simulink model "franka_placement_task_2019b"  (R2019b)
settings: Solver=FixedStepAuto  StartTime=0.0  StopTime=20  FixedStep=0.01  RelTol=1e-3
values from neighbouring files (symbols this model uses):
  a0 = 0.99    [init.m]
  berta = 0.98    [init.m]
  csi = 1    [init.m]
  e_max = 0.01    [init.m]
  F_int_max = 5    [init.m]
  F_max = 2    [init.m]
  g = 9.81    [init.m]
  k_can = 500    [init.m]
  k_shelf = k_table    (= 10000)    [init.m]
  k_table = 10000    [init.m]
  k_wall = k_table    (= 10000)    [init.m]
  l_can = 0.1    [init.m]
  M = 1    [init.m]
  mass = 1    [init.m]
  mass_can = 0.5    [init.m]
  q_max = q_max - deg2rad([0 0 0 10 0 5 0])    [init.m]
  q_min = q_min + deg2rad([0 0 0 10 0 5 0])    [init.m]
  y_can = 0.2    [init.m]
  y_wall = -0.3    [init.m]
  z_shelf = 0.3+0.043    (= 0.343)    [init.m]
  z_table = 0+0.043    (= 0.043)    [init.m]
(part 2 of 2)

== matlab function franka_placement_task_2019b/direct kinematics ==
  data: q_dot input double; q input double; z output double; dz output double; or output
function [z,dz,or] = fcn(q_dot,q)
% persistent dh_c
% if isempty(dh_c)
%     dh_c = Load_Franka_DH();
% end
[DH, Conv] = Load_Franka_DH();
z = zeros(3,1);
%z = get_pos(q);

[p,R] = DirectKinematic(DH,[q;0],Conv);
z = p;
phi = atan2(R(2,1),R(1,1));
teta = atan2(-R(3,1),sqrt(R(3,2)^2 + R(3,3)^2)); 
psi = atan2(R(3,2),R(3,3));
or = [phi teta psi]';

Ja = zeros(3,7);
Ja = get_Jacobianoa(q);

dz = zeros(3,1);
dz = Ja(1:3,1:7)*q_dot;

end

== matlab function franka_placement_task_2019b/PLANNER1/KZ_GENERATOR ==
  settings: updateMethod=DISCRETE  sampleTime=Ts
  data: k output; F_ext input; z input; z_des input; int input; comp input; e_max parameter; F_max parameter; F_int_max parameter
function k = fcn(F_ext, z, z_des, int, comp, e_max, F_max, F_int_max)
%% Description
% Set the K coefficient for a variable impedance controller based on a
% desired trajectory

%% Outputs
% k             stiffness

%% Inputs
% F_ext         measured external force
% z_des         desired trajectory
% z             current position
% int, comp     booleans for the interaction and compensation phase

%% Parameters
% F_int_max     desired interaction force
% F_max         nominal disturbance forces
% e_max         maximum steady-state error

%% persistent initialization
persistent ki kc F_comp int_prec comp_prec z_int z_int_dir 
if isempty(ki)
   ki = F_max/e_max;        % k obtained from interaction
end
if isempty(F_comp)
   F_comp = 0;              % weight to compensate
end
if isempty(kc)
      kc = F_max/e_max;     % k obtained from compensation
end
if isempty(z_int) 
    z_int = 1000;       % obstacle(or interaction) position
end
if isempty(z_int_dir) 
    z_int_dir = 0;          % prohibited direction due to the obstacle
end
if isempty(int_prec)
    int_prec = 0;           % previous values of int
end
if isempty(comp_prec)
    comp_prec = 0;          % previous values od comp
end

%% INTERACTION
% set ki in order to match a desired interaction force with the
% envirorment, and store interaction's position when detected
% X axes
if int == 1
    % detection of an interaction 
    if abs(F_ext-F_comp) > F_max
        if z_int == 1000                     % z_int has not been set yet
            z_int = z;
            z_int_dir = -sign(F_ext-F_comp);
        end
    end
    % setting of ki
    if abs(F_ext-F_comp) > F_int_max 
        % if interaction force is higher than threshold
        if ki*abs(z-z_des) > F_int_max
            ktemp_x = F_int_max/abs(z-z_des);
            if ktemp_x < ki                % ki needs to be only decreased
                ki = ktemp_x;
            end
        end
    end
end

%% COMPENSATION
% set kc in order to compensate the effect of the weight of the object,
% and store it
% X axes
if comp == 1
    % compensation detection
    if z_int == 1000                     % z_int not set before
       if abs(F_ext)/kc > e_max         
            kc = abs(F_ext)/e_max;
            F_comp = F_ext;
       end
    else 
        if z_int_dir == 1                % obstacle in above
            if z < z_int
                if abs(F_ext)/kc > e_max 
                    kc = abs(F_ext)/e_max;
                    F_comp = F_ext;
                end
            end
        else                                % obstacle is below
            if z > z_int
                if abs(F_ext)/kc > e_max
                    kc = abs(F_ext)/e_max;
                    F_comp = F_ext;
                end
            end
        end 
   end
end

%% reset to default values when comp or int shifts to zero
if comp==0 && comp_prec==1
    kc = F_max/e_max;
    F_comp = 0;
end
if int==0 && int_prec==1
    ki = F_max/e_max;
end

%% from int to comp and vice versa
if int==1 && int_prec==0
    if comp_prec == 1
        ki = kc;
    end
    z_int=1000;
    z_int_dir=0;
end
if comp == 1 && comp_prec==0
    if int_prec == 1
        kc = ki;
    end
end

% update to last booleans
int_prec = int;
comp_prec = comp;


%% Selection of Final Values of D-K
% default values
k = abs(F_max)/e_max;

% compensation
if comp == 1
    k = kc;
end

% both compensation and interaction are activated
% if "away" from obstacle set k = kc else ki
if int == 1
    k = ki;
    if comp == 1
        if z_int == 1000
            k = kc;                       % obstacle not reached
        else
            if z_int_dir == 1
                if z_des < z_int
                    k = kc;               % obstacle reached but "going away"
                end
            else
                if z_des > z_int
                    k = kc;               % obstacle reached but "going away"
                end
            end
        end
    else
        if z_int == 1000
            k = F_max/e_max;            % restore to default
        else
            if z_int_dir == 1
                if z_des < z_int
                    k = F_max/e_max;    % restore because "going away"
                end
            else
                if z_des > z_int
                    k = F_max/e_max;    % restore because "going away"
                end
            end
        end
    end
end

end

== matlab function franka_placement_task_2019b/direct kinematics1 ==
  data: q_dot input double; q input double; z output double; dz output double; or output
function [z,dz,or] = fcn(q_dot,q)
coder.extrinsic('get_Ja');
% persistent dh_c
% if isempty(dh_c)
%     dh_c = Load_Franka_DH();
% end
[DH, Conv] = Load_Franka_DH();
z = zeros(3,1);
%z = get_pos(q);

[p,R] = DirectKinematic(DH,[q;0],Conv);
z = p;
phi = atan2(R(2,1),R(1,1));
teta = atan2(-R(3,1),sqrt(R(3,2)^2 + R(3,3)^2)); 
psi = atan2(R(3,2),R(3,3));
or = [phi teta psi]';

Ja = zeros(6,7);
Ja = get_Ja(q);

dz = zeros(3,1);
dz = Ja(1:3,1:7)*q_dot;

end

== matlab function franka_placement_task_2019b/PLANNER/KD_INTERPOLATOR  ==
  settings: updateMethod=DISCRETE  sampleTime=Ts
  data: time input; K output; kx_f input; ky_f input; kz_f input; D output; e_max parameter; F_max parameter; M parameter; berta parameter; a0 parameter; mass parameter; csi parameter
function [K,D] = fcn(time, kx_f, ky_f, kz_f, e_max, F_max, M, berta, a0, mass, csi)
%% Description
% Interpolate K in order to guarantee stability

%% Outputs
% K             Stiffness matrix
% D             Damping matrix

%% Inputs
% kx_f, ky, f   desired values of K

%% Parameters
% F_max         nominal disturbance forces
% e_max         maximum steady-state error
% M             virtual mass
% berta, a0     parameters for the computation of stability conditions
% mass          virtual mass

%% persistent initialization
persistent kx ky kz time_prec
if isempty(time_prec)
    time_prec = 0;              % previous simulation time
end
if isempty(kx)
   kx = F_max/e_max;         % last value of k
end
if isempty(ky)
   ky = F_max/e_max;
end
if isempty(kz)
   kz = F_max/e_max;
end

% set k from desired one 
if kx_f <= kx       
    kx = kx_f;
else 
    % increese k in accordance with the stability conditions
    kx_i = kx;
    k_dotx = berta*(4*a0*sqrt(kx_i/mass)*(kx_i)^(3/2))/(sqrt(kx_i) + 2*a0*csi*sqrt(kx_i));
    k_tempx = kx_i + k_dotx*(time -time_prec);
    if k_tempx > kx_f
        kx = kx_f;
    else
        kx = k_tempx;
    end
end

% Y axes, same as X axes
if ky_f <= ky
    ky = ky_f;
else 
    ky_i = ky;
    k_doty = berta*(4*a0*sqrt(ky_i/mass)*(ky_i)^(3/2))/(sqrt(ky_i) + 2*a0*csi*sqrt(ky_i));
    k_tempy = ky_i + k_doty*(time -time_prec);
    if k_tempy > ky_f
        ky = ky_f;
    else
        ky = k_tempy;
    end
end

% Z axes, same as other axes
if kz_f <= kz
    kz = kz_f;
else 
    kz_i = kz;
    k_dotz = berta*(4*a0*sqrt(kz_i/mass)*(kz_i)^(3/2))/(sqrt(kz_i) + 2*a0*csi*sqrt(kz_i));
    k_tempz = kz_i + k_dotz*(time -time_prec);
    if k_tempz > kz_f
        kz = kz_f;
    else
        kz = k_tempz;
    end
end

time_prec = time;

% damping computation, critically damped condition
dx = sqrt(4*kx*M);
dy = sqrt(4*ky*M);
dz = sqrt(4*kz*M);

%% Final impedance matrices
D = diag([dx, dy, dz]);
K = diag([kx, ky, kz]);

end

== matlab function franka_placement_task_2019b/PLANNER/KX_GENERATOR ==
  settings: updateMethod=DISCRETE  sampleTime=Ts
  data: k output; F_ext input; z input; z_des input; int input; comp input; e_max parameter; F_max parameter; F_int_max parameter
function k = fcn(F_ext, z, z_des, int, comp, e_max, F_max, F_int_max)
%% Description
% Set the K coefficient for a variable impedance controller based on a
% desired trajectory

%% Outputs
% k             stiffness

%% Inputs
% F_ext         measured external force
% z_des         desired trajectory
% z             current position
% int, comp     booleans for the interaction and compensation phase

%% Parameters
% F_int_max     desired interaction force
% F_max         nominal disturbance forces
% e_max         maximum steady-state error

%% persistent initialization
persistent ki kc F_comp int_prec comp_prec z_int z_int_dir 
if isempty(ki)
   ki = F_max/e_max;        % k obtained from interaction
end
if isempty(F_comp)
   F_comp = 0;              % weight to compensate
end
if isempty(kc)
      kc = F_max/e_max;     % k obtained from compensation
end
if isempty(z_int) 
    z_int = 1000;       % obstacle(or interaction) position
end
if isempty(z_int_dir) 
    z_int_dir = 0;          % prohibited direction due to the obstacle
end
if isempty(int_prec)
    int_prec = 0;           % previous values of int
end
if isempty(comp_prec)
    comp_prec = 0;          % previous values od comp
end

%% INTERACTION
% set ki in order to match a desired interaction force with the
% envirorment, and store interaction's position when detected
% X axes
if int == 1
    % detection of an interaction 
    if abs(F_ext-F_comp) > F_max
        if z_int == 1000                     % z_int has not been set yet
            z_int = z;
            z_int_dir = -sign(F_ext-F_comp);
        end
    end
    % setting of ki
    if abs(F_ext-F_comp) > F_int_max 
        % if interaction force is higher than threshold
        if ki*abs(z-z_des) > F_int_max
            ktemp_x = F_int_max/abs(z-z_des);
            if ktemp_x < ki                % ki needs to be only decreased
                ki = ktemp_x;
            end
        end
    end
end

%% COMPENSATION
% set kc in order to compensate the effect of the weight of the object,
% and store it
% X axes
if comp == 1
    % compensation detection
    if z_int == 1000                     % z_int not set before
       if abs(F_ext)/kc > e_max         
            kc = abs(F_ext)/e_max;
            F_comp = F_ext;
       end
    else 
        if z_int_dir == 1                % obstacle in above
            if z < z_int
                if abs(F_ext)/kc > e_max 
                    kc = abs(F_ext)/e_max;
                    F_comp = F_ext;
                end
            end
        else                                % obstacle is below
            if z > z_int
                if abs(F_ext)/kc > e_max
                    kc = abs(F_ext)/e_max;
                    F_comp = F_ext;
                end
            end
        end 
   end
end

%% reset to default values when comp or int shifts to zero
if comp==0 && comp_prec==1
    kc = F_max/e_max;
    F_comp = 0;
end
if int==0 && int_prec==1
    ki = F_max/e_max;
end

%% from int to comp and vice versa
if int==1 && int_prec==0
    if comp_prec == 1
        ki = kc;
    end
    z_int=1000;
    z_int_dir=0;
end
if comp == 1 && comp_prec==0
    if int_prec == 1
        kc = ki;
    end
end

% update to last booleans
int_prec = int;
comp_prec = comp;


%% Selection of Final Values of D-K
% default values
k = abs(F_max)/e_max;

% compensation
if comp == 1
    k = kc;
end

% both compensation and interaction are activated
% if "away" from obstacle set k = kc else ki
if int == 1
    k = ki;
    if comp == 1
        if z_int == 1000
            k = kc;                       % obstacle not reached
        else
            if z_int_dir == 1
                if z_des < z_int
                    k = kc;               % obstacle reached but "going away"
                end
            else
                if z_des > z_int
                    k = kc;               % obstacle reached but "going away"
                end
            end
        end
    else
        if z_int == 1000
            k = F_max/e_max;            % restore to default
        else
            if z_int_dir == 1
                if z_des < z_int
                    k = F_max/e_max;    % restore because "going away"
                end
            else
                if z_des > z_int
                    k = F_max/e_max;    % restore because "going away"
                end
            end
        end
    end
end

end

== matlab function franka_placement_task_2019b/TRAJECTORY/INTERPOLATOR ==
  data: xi input; z_des output; xf input; tf input; t input; v input; alpha input; dz_des output; ddz_des output
function [z_des, dz_des, ddz_des] = fcn(xi, xf, tf, t, v, alpha)

ta = alpha*tf; 
xa = (1/2)*v*ta;

if t >= 0 && t < ta
    ddz_des = v./ta;
    dz_des = ddz_des*t;
    z_des = xi + (1/2)*ddz_des*t^2;
elseif t >= ta && t < (tf-ta)
    ddz_des = [0; 0; 0]; 
    dz_des = v; 
    z_des = xi + xa + dz_des*(t-ta);
elseif t >= (tf- ta) && t < tf
    ddz_des = -v./ta;
    dz_des = v + ddz_des*(t - (tf-ta));
    z_des = xi + xa + v*(tf-2*ta) + v*(t-(tf-ta)) + (1/2)*ddz_des*(t-(tf-ta))^2;
else 
    ddz_des = [0; 0; 0];
    dz_des = [0; 0; 0];
    z_des = xf;
end

end

== matlab function franka_placement_task_2019b/FRANKA_Model_Joint_Space1/GRAVITY ==
  data: q input; G output double
function G = fcn(q)

G = zeros(7,1);
G = get_GravityVector(q);

end

== matlab function franka_placement_task_2019b/FRANKA_Model_Joint_Space1/Joint Friction1 ==
  data: q_dot input; tau_f output
function tau_f = fcn(q_dot)
D=eye(7)*1;
tau_f = -D*q_dot;

end

== matlab function franka_placement_task_2019b/FRANKA_Model_Joint_Space1/Joint Friction ==
  data: q_dot input; tau_f output
function tau_f = fcn(q_dot)

tau_f = get_FrictionTorque(q_dot);

end

== matlab function franka_placement_task_2019b/M_D_S5/DAMPER ==
  data: dx input; y output; D input
function y = fcn(dx, D)
y = - D*dx;
end

== matlab function franka_placement_task_2019b/M_D_S5/MASS^-1 ==
  data: M input; ddx output; F_tot input
function ddx = fcn(M,F_tot)
ddx = (M^-1)*F_tot;


end

== matlab function franka_placement_task_2019b/M_D_S5/SPRING ==
  data: x input; tau output; K input
function tau = fcn(x, K)
tau= -K*x;
end

== matlab function franka_placement_task_2019b/FRANKA_Model_Joint_Space1/MASS^-1 ==
  data: q input; ddq output; F_tot input double
function ddq = fcn(q,F_tot)

B = zeros(7,7);
B = get_MassMatrix(q);

ddq = B\F_tot;                      % Ftot*M^-1

end

== matlab function franka_placement_task_2019b/FRANKA_Model_Joint_Space1/MATLAB Function ==
  data: F input; F_ext output double; q input
function F_ext = fcn(F,q)

Ja = zeros(6,7);
Ja = get_Jacobianoa(q);

F_ext = zeros(7,1);
F_ext = (Ja')*F;

end

== matlab function franka_placement_task_2019b/MATLAB Function ==
  data: K output; D output
function [K, D] = fcn()
K = zeros(6,6);
K(1:3,1:3) = diag([1000 1000 1000]); %Klin
K(4:6,4:6) = diag ([300 300 300]); %Kor
D = zeros(6,6);
D(1:3,1:3) = diag([2*sqrt(1000) 2*sqrt(1000) 2*sqrt(1000)]);
D(4:6,4:6) = diag([2*sqrt(300) 2*sqrt(300) 2*sqrt(300)]);

end

== matlab function franka_placement_task_2019b/CONTROLLER1 ==
  data: F_ext input; Km input; Dm input; or_des input; zdes input; tau output double; dzdes input; ddzdes input; q input; q_dot input; M parameter
function tau = fcn(F_ext, Km, Dm, or_des, zdes, dzdes, ddzdes, q, q_dot, M)
coder.extrinsic('get_MassMatrix','get_Ja_dot','get_Ja','get_GravityVector','get_FrictionTorque','get_CoriolisMatrix')
coder.extrinsic('wrapToPi');
% dz = zeros(2,1);
% z = zeros(2,1);
B = zeros(7,7);
S = zeros(7,7);
G = zeros(7,1);
Ja = zeros(6,7);
Ja_dot = zeros(6,7);
tau_fric = zeros(7,1);
Bm = eye(6)*M;
Ja = get_Ja(q);
Ja(isnan(Ja)) = 1;
% cond_Ja = cond(Ja)
Ja_dot = get_Ja_dot(q,q_dot);
Ja_dot(isnan(Ja_dot)) = 1;

% cond_Ja_dot = cond(Ja_dot)

%% Computation of end-effector's position and orientation 
[DH, Conv] = Load_Franka_DH();
[p,R] = DirectKinematic(DH,[q;0],Conv);
z = zeros(3,1);
%z = get_pos(q);
z = p;
dz = Ja(1:3,1:7)*q_dot;
phi = atan2(R(2,1),R(1,1));
teta = atan2(-R(3,1),sqrt(R(3,2)^2 + R(3,3)^2)); 
psi = atan2(R(3,2),R(3,3));
or = [phi teta psi]';

% pseudoinverse
B = get_MassMatrix(q);
B_inv = inv(B);
B_inv(isnan(B_inv)) = 1;
Ja_inv = B_inv*(Ja')*inv(Ja*B_inv*Ja');
Ja_inv(isnan(Ja_inv)) = 1;

% cond_Ja_inv = cond(Ja_inv)
% cond_B = cond(B)


% Matrices
S = get_CoriolisMatrix(q,q_dot);
tau_fric = get_FrictionTorque(q_dot);
G = get_GravityVector(q);
I = eye(6);

% Impedance controller (De Luca)
%{
Bx = (Ja_inv')* B * Ja_inv;
tau = B*Ja_inv*(ddzdes - Ja_dot*q_dot + ...
    inv(Bm)*(Dm*(dzdes - dz) + Km*(zdes- z))) + S*q_dot + tau_fric + G + ...
    (Ja')*(Bx*inv(Bm) - I)*F_ext;
%}
% Impedance controller (Albu Shaffer)
L = inv(Ja * B_inv * Ja');
L(isnan(L)) = 1;
% cond_L = cond(L)
e_pos = (z - zdes);
e_pos_dot = (dz - dzdes);
%e_or = (or - or_des); 
e_or = zeros(3,1);
e_or = wrapToPi(or-or_des);
e_or_dot = Ja(4:6,1:7)*q_dot;
e = [e_pos; e_or];
e_dot = [e_pos_dot; e_or_dot];                                                                   
a_des = [ddzdes; zeros(3,1)];
F_tau = L*a_des - L*inv(Bm)*(Dm*e_dot + Km*e) + (L*inv(Bm) - I)*F_ext - L*Ja_dot*q_dot;
tau = (Ja')*F_tau + S*q_dot + tau_fric + G;

end

== matlab function franka_placement_task_2019b/FRANKA_Model_Joint_Space2/CORIOLIS ==
  data: q input; Fc output double; q_dot input
function Fc = fcn(q,q_dot)
coder.extrinsic('get_CoriolisMatrix');
C = zeros(7,7);
C = get_CoriolisMatrix(q,q_dot);

Fc = C*q_dot;

end

== matlab function franka_placement_task_2019b/FRANKA_Model_Joint_Space2/GRAVITY ==
  data: q input; G output double
function G = fcn(q)
coder.extrinsic('get_GravityVector');
G = zeros(7,1);
G = get_GravityVector(q);

end

== matlab function franka_placement_task_2019b/FRANKA_Model_Joint_Space2/Joint Friction ==
  data: q_dot input; tau_f output
function tau_f = fcn(q_dot)
coder.extrinsic('get_FrictionTorque');
tau_f = zeros(7,1);
tau_f = get_FrictionTorque(q_dot);

end

== matlab function franka_placement_task_2019b/FRANKA_Model_Joint_Space2/Joint Friction1 ==
  data: q_dot input; tau_f output
function tau_f = fcn(q_dot)
D=eye(7)*1;
tau_f = -D*q_dot;

end

== matlab function franka_placement_task_2019b/FRANKA_Model_Joint_Space2/MASS^-1 ==
  data: q input; ddq output; F_tot input double
function ddq = fcn(q,F_tot)
coder.extrinsic('get_MassMatrix');
B = zeros(7,7);
B = get_MassMatrix(q);

% ddq = B\F_tot;     % Ftot*M^-1

B_inv = inv(B);
B_inv(isnan(B_inv)) = 1;
ddq = B_inv*F_tot;

% B_modello = cond(B)

end

== matlab function franka_placement_task_2019b/FRANKA_Model_Joint_Space2/MATLAB Function ==
  data: F input; F_ext output double; q input
function F_ext = fcn(F,q)
coder.extrinsic('get_Ja');
Ja = zeros(6,7);
Ja = get_Ja(q);

F_ext = zeros(7,1);
F_ext = (Ja')*F;

end

== matlab function franka_placement_task_2019b/F_ext4 ==
  data: z input; F_ext output; grasping input; mass_can parameter; g parameter; phase input; y_can parameter; z_table parameter; k_can parameter; k_table parameter; l_can parameter; y_wall parameter; z_shelf parameter; k_wall parameter; k_shelf parameter
function F_ext = fcn(z, grasping, mass_can, g, phase, y_can, z_table, k_can, k_table, l_can, y_wall, z_shelf, k_wall, k_shelf) 

% hypothesis: table reaction force with elastic behaviour
F_ext = zeros(3,1);
F_ext(1) = 0;
if phase == 1
    % if contact is happened with can
    if grasping == 0
        if z(2) < y_can
            F_ext(2) = -k_can*(z(2) - y_can);    
        end
        if z(3) < z_table
            F_ext(3) = -k_table*(z(3) - z_table);
        end
    else 
        if z(3) < z_table
            F_ext(3) = -k_table*(z(3)-z_table);       
        else 
            if (abs(k_table*(z(3)-z_table)) < abs(mass_can*g))
                F_ext(3) = - k_table*(z(3)-z_table); 
            else 
                F_ext(3) = - mass_can*g;
            end    
        end
    end
elseif phase == 2
    if z(2) < y_wall + l_can
        F_ext(2) = -k_wall*(z(2) - (l_can + y_wall));
    end
    if z(3) < z_shelf
        F_ext(3) = -k_shelf*(z(3) - z_shelf);
    else 
        if (abs(k_shelf*(z(3)-z_shelf)) < abs(mass_can*g))
            F_ext(3) = - k_shelf*(z(3)-z_shelf); 
        else 
            F_ext(3) = - mass_can*g;
        end 
    end
else
    if z(2) < y_wall + l_can
        F_ext(2) = -k_wall*(z(2) - (l_can + y_wall));
    end
    if z(3) < z_shelf
        F_ext(3) = -k_shelf*(z(3) - z_shelf);
    end
end

== matlab function franka_placement_task_2019b/PLANNER2/KY_GENERATOR ==
  settings: updateMethod=DISCRETE  sampleTime=Ts
  data: k output; F_ext input; z input; z_des input; dz_des input; int input; comp input; e_max parameter; F_max parameter; F_int_max parameter
function k = fcn(F_ext, z, z_des, dz_des, int, comp, e_max, F_max, F_int_max)
%% Description
% Set the K coefficient for a variable impedance controller based on a
% desired trajectory

%% Outputs
% k             stiffness

%% Inputs
% F_ext         measured external force
% z_des         desired trajectory
% z             current position
% int, comp     booleans for the interaction and compensation phase

%% Parameters
% F_int_max     desired interaction force
% F_max         nominal disturbance forces
% e_max         maximum steady-state error

%% persistent initialization
persistent ki kc F_comp int_prec comp_prec z_int z_int_dir set_F_comp
if isempty(ki)
   ki = F_max/e_max;        % k obtained from interaction
end
if isempty(F_comp)
   F_comp = 0;              % weight to compensate
end
if isempty(kc)
      kc = F_max/e_max;     % k obtained from compensation
end
if isempty(z_int) 
    z_int = 1000;       % obstacle(or interaction) position
end
if isempty(z_int_dir) 
    z_int_dir = 0;          % prohibited direction due to the obstacle
end
if isempty(int_prec)
    int_prec = 0;           % previous values of int
end
if isempty(comp_prec)
    comp_prec = 0;          % previous values od comp
end
if isempty(set_F_comp)
    set_F_comp = 1;
end
%% INTERACTION
% set ki in order to match a desired interaction force with the
% envirorment, and store interaction's position when detected
% X axes
if int == 1
    % detection of an interaction 
    if abs(F_ext-F_comp) > F_max
        if z_int == 1000                     % z_int has not been set yet
            z_int = z;
            z_int_dir = -sign(F_ext-F_comp);
            set_F_comp = 0; 
        end
    end
    % setting of ki
    if abs(F_ext-F_comp) > F_int_max 
        % if interaction force is higher than threshold
        if ki*abs(z-z_des) > F_int_max
            ktemp_x = F_int_max/abs(z-z_des);
            if ktemp_x < ki                % ki needs to be only decreased
                ki = ktemp_x;
            end
        end
    end
end

%% COMPENSATION
% set kc in order to compensate the effect of the weight of the object,
% and store it
% X axes
if comp == 1
    % compensation detection
    if z_int == 1000                     % z_int not set before
        if abs(F_ext)/kc > e_max         
            kc = abs(F_ext)/e_max;
            if set_F_comp > 0.1
                F_comp = F_ext;
            end
        end
    else 
        if z_int_dir == 1                % obstacle in above
            if z < z_int
                if abs(F_ext)/kc > e_max 
                    kc = abs(F_ext)/e_max;
                    if set_F_comp > 0.1
                        F_comp = F_ext;
                    end
                end
            end
        else                                % obstacle is below
            if z > z_int
                if abs(F_ext)/kc > e_max
                    kc = abs(F_ext)/e_max;
                    if set_F_comp > 0.1
                        F_comp = F_ext;
                    end
                end
            end
        end 
   end
end

%% reset to default values when comp or int shifts to zero
if comp==0 && comp_prec==1
    kc = F_max/e_max;
    F_comp = 0;
    set_F_comp = 0;
end
if int==0 && int_prec==1
    ki = F_max/e_max;
end

%% from int to comp and vice versa
if int==1 && int_prec==0
    if comp_prec == 1
        ki = kc;
    end
    z_int=1000;
    z_int_dir=0;
end
if comp == 1 && comp_prec==0
    if int_prec == 1
        kc = ki;
    end
    set_F_comp = 1;
end

% update to last booleans
int_prec = int;
comp_prec = comp;


%% Selection of Final Values of D-K
% default values
k = abs(F_max)/e_max;

% compensation
if comp == 1
    k = kc;
end

% both compensation and interaction are activated
% if "away" from obstacle set k = kc else ki
if int == 1
    k = ki;
    if comp == 1
        if z_int == 1000
            k = kc;                       % obstacle not reached
        else
            if z_int_dir == 1
                if z_des < z_int
                    if sign(dz_des*z_int_dir) < 0
                        k = kc;               % obstacle reached but "going away"
                    end
                end
            else
                if z_des > z_int
                    if sign(dz_des*z_int_dir) < 0
                        k = kc;               % obstacle reached but "going away"
                    end
                end
            end
        end
    else
        if z_int == 1000
            k = F_max/e_max;            % restore to default
        else
            if z_int_dir == 1
                if z_des < z_int
                    k = F_max/e_max;    % restore because "going away"
                end
            else
                if z_des > z_int
                    k = F_max/e_max;    % restore because "going away"
                end
            end
        end
    end
end

end

== matlab function franka_placement_task_2019b/PLANNER2/KD_INTERPOLATOR  ==
  settings: updateMethod=DISCRETE  sampleTime=Ts
  data: time input; K output; kx_f input; ky_f input; kz_f input; D output; e_max parameter; F_max parameter; M parameter; berta parameter; a0 parameter; mass parameter; csi parameter; Kvis output; Dvis output
function [K,D,Kvis, Dvis] = fcn(time, kx_f, ky_f, kz_f, e_max, F_max, M, berta, a0, mass, csi)
%% Description
% Interpolate K in order to guarantee stability

%% Outputs
% K             Stiffness matrix
% D             Damping matrix

%% Inputs
% kx_f, ky, f   desired values of K

%% Parameters
% F_max         nominal disturbance forces
% e_max         maximum steady-state error
% M             virtual mass
% berta, a0     parameters for the computation of stability conditions
% mass          virtual mass

%% persistent initialization
persistent kx ky kz time_prec
if isempty(time_prec)
    time_prec = 0;              % previous simulation time
end
if isempty(kx)
   kx = F_max/e_max;         % last value of k
end
if isempty(ky)
   ky = F_max/e_max;
end
if isempty(kz)
   kz = F_max/e_max;
end

% set k from desired one 
if kx_f <= kx       
    kx = kx_f;
else 
    % increese k in accordance with the stability conditions
    kx_i = kx;
    k_dotx = berta*(4*a0*sqrt(kx_i/mass)*(kx_i)^(3/2))/(sqrt(kx_i) + 2*a0*csi*sqrt(kx_i));
    k_tempx = kx_i + k_dotx*(time -time_prec);
    if k_tempx > kx_f
        kx = kx_f;
    else
        kx = k_tempx;
    end
end

% Y axes, same as X axes
if ky_f <= ky
    ky = ky_f;
else 
    ky_i = ky;
    k_doty = berta*(4*a0*sqrt(ky_i/mass)*(ky_i)^(3/2))/(sqrt(ky_i) + 2*a0*csi*sqrt(ky_i));
    k_tempy = ky_i + k_doty*(time -time_prec);
    if k_tempy > ky_f
        ky = ky_f;
    else
        ky = k_tempy;
    end
end

% Z axes, same as other axes
if kz_f <= kz
    kz = kz_f;
else 
    kz_i = kz;
    k_dotz = berta*(4*a0*sqrt(kz_i/mass)*(kz_i)^(3/2))/(sqrt(kz_i) + 2*a0*csi*sqrt(kz_i));
    k_tempz = kz_i + k_dotz*(time -time_prec);
    if k_tempz > kz_f
        kz = kz_f;
    else
        kz = k_tempz;
    end
end

time_prec = time;

% damping computation, critically damped condition
dx = sqrt(4*kx*M);
dy = sqrt(4*ky*M);
dz = sqrt(4*kz*M);

%% Final impedance matrices
D = zeros(6,6);
K = zeros(6,6);
D(1:3,1:3) = diag([dx, dy, dz]);
D(4:6,4:6) = diag([2*sqrt(300) 2*sqrt(300) 2*sqrt(300)]); %rot damping
K(1:3,1:3) = diag([kx, ky, kz]);
K(4:6,4:6) = diag ([300 300 300]); %rot stiffness
Kvis = [kx; ky; kz];
Dvis = [dx; dy; dz];
end

== matlab function franka_placement_task_2019b/PLANNER2/KX_GENERATOR ==
  settings: updateMethod=DISCRETE  sampleTime=Ts
  data: k output; F_ext input; z input; z_des input; dz_des input; int input; comp input; e_max parameter; F_max parameter; F_int_max parameter
function k = fcn(F_ext, z, z_des, dz_des, int, comp, e_max, F_max, F_int_max)
%% Description
% Set the K coefficient for a variable impedance controller based on a
% desired trajectory

%% Outputs
% k             stiffness

%% Inputs
% F_ext         measured external force
% z_des         desired trajectory
% z             current position
% int, comp     booleans for the interaction and compensation phase

%% Parameters
% F_int_max     desired interaction force
% F_max         nominal disturbance forces
% e_max         maximum steady-state error

%% persistent initialization
persistent ki kc F_comp int_prec comp_prec z_int z_int_dir set_F_comp
if isempty(ki)
   ki = F_max/e_max;        % k obtained from interaction
end
if isempty(F_comp)
   F_comp = 0;              % weight to compensate
end
if isempty(kc)
      kc = F_max/e_max;     % k obtained from compensation
end
if isempty(z_int) 
    z_int = 1000;       % obstacle(or interaction) position
end
if isempty(z_int_dir) 
    z_int_dir = 0;          % prohibited direction due to the obstacle
end
if isempty(int_prec)
    int_prec = 0;           % previous values of int
end
if isempty(comp_prec)
    comp_prec = 0;          % previous values od comp
end
if isempty(set_F_comp)
    set_F_comp = 1;
end
%% INTERACTION
% set ki in order to match a desired interaction force with the
% envirorment, and store interaction's position when detected
% X axes
if int == 1
    % detection of an interaction 
    if abs(F_ext-F_comp) > F_max
        if z_int == 1000                     % z_int has not been set yet
            z_int = z;
            z_int_dir = -sign(F_ext-F_comp);
            set_F_comp = 0; 
        end
    end
    % setting of ki
    if abs(F_ext-F_comp) > F_int_max 
        % if interaction force is higher than threshold
        if ki*abs(z-z_des) > F_int_max
            ktemp_x = F_int_max/abs(z-z_des);
            if ktemp_x < ki                % ki needs to be only decreased
                ki = ktemp_x;
            end
        end
    end
end

%% COMPENSATION
% set kc in order to compensate the effect of the weight of the object,
% and store it
% X axes
if comp == 1
    % compensation detection
    if z_int == 1000                     % z_int not set before
        if abs(F_ext)/kc > e_max         
            kc = abs(F_ext)/e_max;
            if set_F_comp > 0.1
                F_comp = F_ext;
            end
        end
    else 
        if z_int_dir == 1                % obstacle in above
            if z < z_int
                if abs(F_ext)/kc > e_max 
                    kc = abs(F_ext)/e_max;
                    if set_F_comp > 0.1
                        F_comp = F_ext;
                    end
                end
            end
        else                                % obstacle is below
            if z > z_int
                if abs(F_ext)/kc > e_max
                    kc = abs(F_ext)/e_max;
                    if set_F_comp > 0.1
                        F_comp = F_ext;
                    end
                end
            end
        end 
   end
end

%% reset to default values when comp or int shifts to zero
if comp==0 && comp_prec==1
    kc = F_max/e_max;
    F_comp = 0;
    set_F_comp = 0;
end
if int==0 && int_prec==1
    ki = F_max/e_max;
end

%% from int to comp and vice versa
if int==1 && int_prec==0
    if comp_prec == 1
        ki = kc;
    end
    z_int=1000;
    z_int_dir=0;
end
if comp == 1 && comp_prec==0
    if int_prec == 1
        kc = ki;
    end
    set_F_comp = 1;
end

% update to last booleans
int_prec = int;
comp_prec = comp;


%% Selection of Final Values of D-K
% default values
k = abs(F_max)/e_max;

% compensation
if comp == 1
    k = kc;
end

% both compensation and interaction are activated
% if "away" from obstacle set k = kc else ki
if int == 1
    k = ki;
    if comp == 1
        if z_int == 1000
            k = kc;                       % obstacle not reached
        else
            if z_int_dir == 1
                if z_des < z_int
                    if sign(dz_des*z_int_dir) < 0
                        k = kc;               % obstacle reached but "going away"
                    end
                end
            else
                if z_des > z_int
                    if sign(dz_des*z_int_dir) < 0
                        k = kc;               % obstacle reached but "going away"
                    end
                end
            end
        end
    else
        if z_int == 1000
            k = F_max/e_max;            % restore to default
        else
            if z_int_dir == 1
                if z_des < z_int
                    k = F_max/e_max;    % restore because "going away"
                end
            else
                if z_des > z_int
                    k = F_max/e_max;    % restore because "going away"
                end
            end
        end
    end
end

end

== matlab function franka_placement_task_2019b/PLANNER2/KZ_GENERATOR ==
  settings: updateMethod=DISCRETE  sampleTime=Ts
  data: k output; F_ext input; z input; z_des input; dz_des input; int input; comp input; e_max parameter; F_max parameter; F_int_max parameter
function k = fcn(F_ext, z, z_des, dz_des, int, comp, e_max, F_max, F_int_max)
%% Description
% Set the K coefficient for a variable impedance controller based on a
% desired trajectory

%% Outputs
% k             stiffness

%% Inputs
% F_ext         measured external force
% z_des         desired trajectory
% z             current position
% int, comp     booleans for the interaction and compensation phase

%% Parameters
% F_int_max     desired interaction force
% F_max         nominal disturbance forces
% e_max         maximum steady-state error

%% persistent initialization
persistent ki kc F_comp int_prec comp_prec z_int z_int_dir set_F_comp
if isempty(ki)
   ki = F_max/e_max;        % k obtained from interaction
end
if isempty(F_comp)
   F_comp = 0;              % weight to compensate
end
if isempty(kc)
      kc = F_max/e_max;     % k obtained from compensation
end
if isempty(z_int) 
    z_int = 1000;       % obstacle(or interaction) position
end
if isempty(z_int_dir) 
    z_int_dir = 0;          % prohibited direction due to the obstacle
end
if isempty(int_prec)
    int_prec = 0;           % previous values of int
end
if isempty(comp_prec)
    comp_prec = 0;          % previous values od comp
end
if isempty(set_F_comp)
    set_F_comp = 1;
end
%% INTERACTION
% set ki in order to match a desired interaction force with the
% envirorment, and store interaction's position when detected
% X axes
if int == 1
    % detection of an interaction 
    if abs(F_ext-F_comp) > F_max
        if z_int == 1000                     % z_int has not been set yet
            z_int = z;
            z_int_dir = -sign(F_ext-F_comp);
            set_F_comp = 0; 
        end
    end
    % setting of ki
    if abs(F_ext-F_comp) > F_int_max 
        % if interaction force is higher than threshold
        if ki*abs(z-z_des) > F_int_max
            ktemp_x = F_int_max/abs(z-z_des);
            if ktemp_x < ki                % ki needs to be only decreased
                ki = ktemp_x;
            end
        end
    end
end

%% COMPENSATION
% set kc in order to compensate the effect of the weight of the object,
% and store it
% X axes
if comp == 1
    % compensation detection
    if z_int == 1000                     % z_int not set before
        if abs(F_ext)/kc > e_max         
            kc = abs(F_ext)/e_max;
            if set_F_comp > 0.1
                F_comp = F_ext;
            end
        end
    else 
        if z_int_dir == 1                % obstacle in above
            if z < z_int
                if abs(F_ext)/kc > e_max 
                    kc = abs(F_ext)/e_max;
                    if set_F_comp > 0.1
                        F_comp = F_ext;
                    end
                end
            end
        else                                % obstacle is below
            if z > z_int
                if abs(F_ext)/kc > e_max
                    kc = abs(F_ext)/e_max;
                    if set_F_comp > 0.1
                        F_comp = F_ext;
                    end
                end
            end
        end 
   end
end

%% reset to default values when comp or int shifts to zero
if comp==0 && comp_prec==1
    kc = F_max/e_max;
    F_comp = 0;
    set_F_comp = 0;
end
if int==0 && int_prec==1
    ki = F_max/e_max;
end

%% from int to comp and vice versa
if int==1 && int_prec==0
    if comp_prec == 1
        ki = kc;
    end
    z_int=1000;
    z_int_dir=0;
end
if comp == 1 && comp_prec==0
    if int_prec == 1
        kc = ki;
    end
    set_F_comp = 1;
end

% update to last booleans
int_prec = int;
comp_prec = comp;


%% Selection of Final Values of D-K
% default values
k = abs(F_max)/e_max;

% compensation
if comp == 1
    k = kc;
end

% both compensation and interaction are activated
% if "away" from obstacle set k = kc else ki
if int == 1
    k = ki;
    if comp == 1
        if z_int == 1000
            k = kc;                       % obstacle not reached
        else
            if z_int_dir == 1
                if z_des < z_int
                    if sign(dz_des*z_int_dir) < 0
                        k = kc;               % obstacle reached but "going away"
                    end
                end
            else
                if z_des > z_int
                    if sign(dz_des*z_int_dir) < 0
                        k = kc;               % obstacle reached but "going away"
                    end
                end
            end
        end
    else
        if z_int == 1000
            k = F_max/e_max;            % restore to default
        else
            if z_int_dir == 1
                if z_des < z_int
                    k = F_max/e_max;    % restore because "going away"
                end
            else
                if z_des > z_int
                    k = F_max/e_max;    % restore because "going away"
                end
            end
        end
    end
end

end

== matlab function franka_placement_task_2019b/direct kinematics2 ==
  data: q_dot input double; q input double; z output double; dz output double; or output
function [z,dz,or] = fcn(q_dot,q)
coder.extrinsic('get_Ja');
% persistent dh_c
% if isempty(dh_c)
%     dh_c = Load_Franka_DH();
% end
[DH, Conv] = Load_Franka_DH();
z = zeros(3,1);
%z = get_pos(q);

[p,R] = DirectKinematic(DH,[q;0],Conv);
z = p;
phi = atan2(R(2,1),R(1,1));
teta = atan2(-R(3,1),sqrt(R(3,2)^2 + R(3,3)^2)); 
psi = atan2(R(3,2),R(3,3));
or = [phi teta psi]';

Ja = zeros(6,7);
Ja = get_Ja(q);

dz = zeros(3,1);
dz = Ja(1:3,1:7)*q_dot;

end

== matlab function franka_placement_task_2019b/null_space_controller1 ==
  data: q input; tau output; q_dot input
function tau = nsc(q, q_dot)
coder.extrinsic('get_Ja','get_MassMatrix');
Ja = zeros(6,7);
B = zeros(7,7);
q_min = [-2.8973   -1.7628   -2.8973   -3.0718   -2.8973   -0.0175  -2.8973];
q_min = q_min + deg2rad([0 0 0 10 0 5 0]);
%        166.0031  101.0010  166.0031 -3.9992   166.0031   215.0024  166.0031
q_max = [ 2.8973    1.7628    2.8973  -0.0698    2.8973    3.7525    2.8973];
q_max = q_max - deg2rad([0 0 0 10 0 5 0]);

q_des = (q_max + q_min)'/2;

Ja = get_Ja(q);
Ja(isnan(Ja)) = 1;
B = get_MassMatrix(q);
B_inv = inv(B);
B_inv(isnan(B_inv)) = 1;
%Ja_inv = inv(B)*(Ja')*inv(Ja*inv(B)*Ja');
Ja_t_inv = inv(Ja*B_inv*Ja')*Ja*B_inv; %inertia-weighted pseudo inverse Ja'
Ja_t_inv(isnan(Ja_t_inv)) = 1;
% cond_Ja_t_inv = cond(Ja_t_inv)

Ja_inv = Ja_t_inv'; 
% add joint friction
D_joints = eye(7)*2;
K_joints = eye(7)*10;
%N = eye(7) - Ja_inv*Ja;
N = eye(7) - Ja'*(Ja_t_inv);
tau = N*(K_joints*(q_des - q) -D_joints*q_dot);

end
